simulink library "hostLogic"  (R2014b)
settings: Solver=ode45  StartTime=0.0  StopTime=10.0  RelTol=1e-3
libraries: minionLogic x2
settings Model: Creator=scastro  LastModifiedBy=scastro

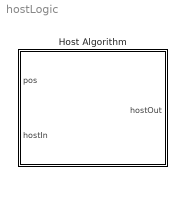
== system hostLogic ==
  Host Algorithm : Stateflow chart  TreatAsAtomicUnit=on

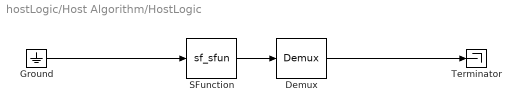
== system hostLogic/Host Algorithm/HostLogic ==
  " Demux " : Demux  Outputs=1
  " Ground " : Ground
  " SFunction " : S-Function  Tag=Stateflow S-Function hostLib 1  FunctionName=sf_sfun  PortCounts=[1 1]  EnableBusSupport=off
  " Terminator " : Terminator
  wires:
  " Ground "/1 -> " SFunction "/1
  " Demux "/1 -> " Terminator "/1
  " SFunction "/1 -> " Demux "/1

== stateflow chart hostLogic/Host Algorithm/HostLogic ==
  note: Host related logic
  state Standby
  (default) -> Standby

== stateflow chart hostLogic/Host Algorithm ==
  state ZumoBot [parallel]
    settings: executionOrder=2
  state Sphero [parallel]
    settings: executionOrder=3
  state HostLogic [parallel]
    settings: executionOrder=1
  data: pos input; hostIn input; hostOut output
